simulink model "GFL_SMIB_Scan_LF_Investigation"  (R2024b)
settings: Solver=FixedStepAuto  StartTime=0  StopTime=200  FixedStep=Ts  RelTol=1e-3
PreLoadFcn:
  | FS_Frequency=csvread('Frequency_Sweep.csv',1,0); run lpf_param.m;
InitFcn:
  | FS_Frequency=csvread('Frequency_Sweep.csv',1,0); run lpf_param.m;
StartFcn:
  | FS_Frequency=csvread('Frequency_Sweep.csv',1,0); run lpf_param.m;
StopFcn:
  | run Bode_Draw.m
values from neighbouring files (symbols this model uses):
  D = zeros(6,4)    [TheoreticalImpedancePlot.m]    (also in TheoreticalImpedancePlotGFL.m = zeros(5,4))
  Fbase = 50    [lpf_param.m]
  fpll = 0.1    [lpf_param.m]
  k_lpf = 0.707    [lpf_param.m]
  wc_lpf = 2*pi*fc_lpf    (= 0.628318530718)    [lpf_param.m]
  x_e = [i_d; i_q; i_d_i; i_q_i; v_d_i; v_q_i; theta; v_dc; v_dc_i; i; i_i; v_lk; p_sum_i; p_lk_i]    [InterlinkAcDcB2B.m]
undefined symbols (not defined in the file or in its folder): ApparatusDiscreDamping, ApparatusPara, ApparatusPowerFlow, ApparatusType, DiscIntNeverNeededParam, OtherInputs, PowerFlow, Sbase, Ts, Vbase, Wbase, Ybase, Zbase
libraries: SimplusGT x10, discretizing x8, dspindex x4, spsGroundLib x3, simulink x3, spsControlledCurrentSourceLib x3, spsCurrentMeasurementLib x3, spsVoltageMeasurementLib x3, spsControlledVoltageSourceLib x3, spsThreePhaseSeriesRLCBranchLib x2, dspsnks4 x2, spsThreePhaseVIMeasurementLib x2
(part 2 of 2)

== matlab function GFL_SMIB_Scan_LF_Investigation/Frequency_Sweep/Frequency Sweep ==
  data: EN input; Perturb_DQ output; ResponseDQ input size=[1 6]; FreqSet input; FreqTest input; OutAmp input; Fs input; AmpGain input; xD input; FSResult output; FreqPoint output; RecordTrigger output; xD1 output; End output; CycleEnd output
function [Perturb_DQ, FSResult, FreqPoint, RecordTrigger, xD1, End, CycleEnd] = fcn(EN,ResponseDQ, FreqSet, FreqTest, OutAmp, Fs, AmpGain, xD)
% This function performs online frequency scanning using a state machine. 
%   - D and Q axis perturbations at specified frequencies
%   - The system response measured (Voltage and Currents)
%   - System admittance, Apparatus Admittance and Grid admittance are
%   calculated
% This current version uses a fixed window to detect whether steady state
% has been reached for each frequency point.
%
% Inputs:
%   EN          : Enable signal (1 to run, 0 to reset)
%   ResponseDQ  : 1x6 vector of system responses [ID, IQ, VAD, VAQ, VGD, VGQ]
%   FreqSet     : Vector of frequencies to apply perturbation (Hz)
%   FreqTest    : Vector of frequencies to analyze (DFT) (Hz)
%   OutAmp      : Vector of perturbation amplitudes for each frequency
%   Fs          : Sampling frequency (Hz)
%   AmpGain     : Global gain for perturbation amplitude
%   xD          : State vector (storage between calls)
%
% Outputs:
%   Perturb_DQ    : [OutVD, OutVQ] perturbation signal to inject
%   FSResult      : 2x6 complex vector of 2x2 admittances [Ysys, YA, YG]
%   FreqPoint     : The current frequency being tested
%   RecordTrigger : A one-sample pulse (==1) when a new result is calculated
%   xD1           : Updated state vector for the next time step
%   End           : Boolean Simulation End 
%
% ------------------- Tuning: Steady-state detector ---------------------- %
% These parameters control the sensitivity and speed of the steady-state detector.
MIN_CYCLES_WINDOWS = 1;    % always do at least one full test cycle before checking
MAX_CYCLES_WINDOWS = 20;   % safety cap to avoid hanging if state never stabilizes
TOL_MAG    = 1e-3;         % relative magnitude tolerance for steady-state (0.1%)
TOL_PHASE  = 1*pi/180;     % phase tolerance (radians) (~1 deg)
STABLE_K   = 1;            % consecutive stable cycles required to confirm steady state
EPS        = 1e-12;        % small number to prevent division by zero
CYCLES = 5;                % number of cycles to use for each fixed DFT window
% -------------------Initialise Outputs-----------------------------------%
% Pre-allocate output matrices for admittances
YA        = complex(zeros(2,2)); % Admittance YA = -I / VA
YG        = complex(zeros(2,2)); % Admittance YG = I / VG
Ysys      = complex(zeros(2,2)); % System Admittance Ysys = I / V_perturb
FSResult  = complex(zeros(2,6)); % Final result matrix [Ysys, YA, YG]
RecordTrigger = 0;               % Output trigger pulse
End = 0;                         % Simulation End Boolean
CycleEnd = 0;
% ------------------- Read States ----------------------------------------%
% 'xD' stores the function's internal state between simulation steps.
CaseK = xD(1);    % Current state in the state machine (0, 1, 2, 3, 9)
Ns    = xD(2);    % Number of samples for perturbation signal generation
Nt    = xD(3);    % Number of samples for DFT analysis window
n     = xD(4);    % Current sample counter within a window (1 to Nt)
kc    = xD(5);    % Current frequency index (points to FreqSet(kc))
OutVD = xD(6);    % Current D-axis perturbation output
OutVQ = xD(7);    % Current Q-axis perturbation output
% Sums for DFT accumulation [ID, IQ, VAD, VAQ, VGD, VGQ]
% These are complex accumulators for the 6 response signals.
Sum = complex([xD(8)+1i*xD(9),  xD(10)+1i*xD(11), ...
               xD(20)+1i*xD(21), xD(22)+1i*xD(23), ...
               xD(32)+1i*xD(33), xD(34)+1i*xD(35)]);
% Final DFT results after D-axis sweep [ID, IQ, VAD, VAQ, VGD, VGQ]
FinalD = complex([xD(12)+1i*xD(13),  xD(14)+1i*xD(15), ...
                  xD(24)+1i*xD(25),  xD(26)+1i*xD(27), ...
                  xD(36)+1i*xD(37),  xD(38)+1i*xD(39)]).'; % Transpose to 6x1
% Final DFT results after Q-axis sweep [ID, IQ, VAD, VAQ, VGD, VGQ]
FinalQ = complex([xD(16)+1i*xD(17),  xD(18)+1i*xD(19), ...
                  xD(28)+1i*xD(29),  xD(30)+1i*xD(31), ...
                  xD(40)+1i*xD(41),  xD(42)+1i*xD(43)]).'; % Transpose to 6x1
% --- Legacy TWait(44) removed ---
% Steady-state detector states (shifted down by 1)
cycCount     = xD(44);     % Number of test cycles completed at this frequency
stableCount  = xD(45);     % Number of consecutive stable cycles
PrevRe       = [xD(46) xD(47) xD(48) xD(49) xD(50) xD(51)]; % Real part of previous DFT
PrevIm       = [xD(52) xD(53) xD(54) xD(55) xD(56) xD(57)]; % Imag part of previous DFT
Prev         = complex(PrevRe(:), PrevIm(:));   % 6x1 complex vector of previous DFT results
% Get total number of frequencies to test
FrequencyNum = numel(FreqSet);
% --- Safety Check ---
% Ensure gain is not zero, which would cause division by zero later
if AmpGain==0 || (kc>=1 && kc<=FrequencyNum && OutAmp(kc)==0)
    error('AmpGain and OutAmp(kc) must be non-zero');
end
% Reshape response input to a 1x6 row vector for easier matrix math
Resp = reshape(ResponseDQ,1,6);

%% Main Loop
if EN==0
    % If Enable is low, reset the perturbation outputs
    OutVD=0;
    OutVQ=0;
    % Note: State variables are NOT reset here, they are reset in Case 0
    % when EN goes high.
else
    % --- State Machine ---
    switch CaseK
        case 0  % State 0: Initialization
            RecordTrigger = 0; % Ensure trigger is low
            kc = 1;            % Start with the first frequency
            CaseK = 1;         % Move to setup state
            CycleEnd = 0;
        case 1  % State 1: Setup for new frequency
            if kc > FrequencyNum
                % If frequency index is past the end of the list, sweep is done
                OutVD=0; OutVQ=0; % Turn off perturbation
                CaseK = 9;       % Move to 'finished' state
            else
                % --- Prepare for a new frequency sweep ---
                Sum(:)=0;  % Reset DFT accumulators
                % Calculate number of samples for perturbation generation (Ns)
                % and DFT analysis (Nt) based on Fs, Freq, and CYCLES
                Ns = max(1, round(Fs/FreqSet(kc)*CYCLES));
                Nt = max(1, round(Fs/FreqTest(kc)*CYCLES));
                OutVD=0; OutVQ=0; % Ensure perturbation is off during setup
                n = 1;            % Reset sample counter
                % Reset steady-state detector variables
                cycCount = 0;
                stableCount = 0;
                Prev(:) = 0;
                CaseK = 2;         % Move to D-axis perturbation state
            end
        case 2   % State 2: D-axis perturbation and analysis
            % Generate D-axis sinusoidal perturbation
            OutVD = OutAmp(kc)*sin(2*pi*CYCLES*n/Ns)*AmpGain;
            OutVQ = 0;
            % Calculate DFT complex phasor for this sample
            ang = 2*pi*CYCLES*(n-1)/Nt;
            ph  = sin(ang) + 1i*cos(ang);
            % Accumulate the DFT sum (dot product of response and phasor)
            % % --------- Hanning window weight for this sample ---------
            % if Nt > 1
            %     w_n = 0.5 - 0.5*cos(2*pi*(n-1)/(Nt-1));
            % else
            %     w_n = 1;
            % end
            % Resp_w = Resp * w_n;
            % 
            % % Accumulate the DFT sum (windowed)
            % Sum = Sum + Resp_w * ph;
            Sum = Sum + Resp * ph;
            if n < Nt
                % If window is not full, increment sample counter
                n = n + 1;
            else
                % --- One test cycle completed on D-axis ---
                % Scale the accumulated sum to get the DFT phasor
                scale  = 2*FreqSet(kc)/CYCLES/Fs; % DFT scaling factor
                Curr   = scale*Sum.';     % 6x1 complex phasor result
                if cycCount >= 1
                    % --- Steady-State Check (if not the first cycle) ---
                    % Compare current result (Curr) vs. previous (Prev)
                    % Calculate relative magnitude difference
                    dmag   = abs(abs(Curr) - abs(Prev)) ./ max(abs(Curr), EPS);
                    % Calculate phase difference
                    dphase = angle(Curr) - angle(Prev);
                    % Wrap phase difference to [-pi, pi]
                    dphase = atan2(sin(dphase), cos(dphase));
                    % Check if all 6 signals are stable within tolerance
                    isStable = all(dmag <= TOL_MAG) && all(abs(dphase) <= TOL_PHASE);
                    if isStable
                        stableCount = stableCount + 1; % Increment stable counter
                    else
                        stableCount = 0; % Reset if any signal is unstable
                    end
                end
                Prev      = Curr;         % Store current result for next comparison
                cycCount  = cycCount + 1; % Increment total cycle counter
                % --- Decision: Move on or repeat? ---
                if (cycCount >= MIN_CYCLES_WINDOWS && stableCount >= STABLE_K) || (cycCount >= MAX_CYCLES_WINDOWS)
                    % Condition 1: Min cycles done AND stable count reached
                    % Condition 2: Max cycles limit reached

                    % Accept this result as steady-state for D-axis
                    FinalD = Prev;
                    % Prepare for Q-axis sweep
                    Sum(:) = 0; n = 1; % Reset accumulators and counter
                    cycCount = 0; stableCount = 0; % Reset detector
                    Prev(:)  = 0;
                    CaseK = 3;         % Move to Q-axis state
                    CycleEnd = 1;
                else
                    % Not stable yet, run another test cycle
                    Sum(:) = 0; n = 1;   % Reset for another D-axis cycle
                    % Stay in CaseK = 2
                end
            end
        case 3   % State 3: Q-axis perturbation and analysis
            % This state is analogous to Case 2, but for the Q-axis.
            CycleEnd = 0;
            OutVD = 0;
            OutVQ = OutAmp(kc)*sin(2*pi*CYCLES*n/Ns)*AmpGain;
            % Calculate DFT complex phasor
            ang = 2*pi*CYCLES*(n-1)/Nt;
            ph  = sin(ang) + 1i*cos(ang);
            % Accumulate the DFT sum (dot product of response and phasor)
            % % --------- Hanning window weight for this sample ---------
            % if Nt > 1
            %     w_n = 0.5 - 0.5*cos(2*pi*(n-1)/(Nt-1));
            % else
            %     w_n = 1;
            % end
            % Resp_w = Resp * w_n;

            % Accumulate the DFT sum (windowed)
            % Sum = Sum + Resp_w * ph;
            Sum = Sum + Resp * ph;
            if n < Nt
                % If window is not full, increment sample counter
                n = n + 1;
            else
                % --- One test cycle completed on Q-axis ---
                scale  = 2*FreqSet(kc)/CYCLES/Fs; % DFT scaling
                Curr   = scale*Sum.';     % 6x1 complex phasor
                % --- Steady-State Check ---
                if cycCount >= 1
                    dmag   = abs(abs(Curr) - abs(Prev)) ./ max(abs(Curr), EPS);
                    dphase = angle(Curr) - angle(Prev);
                    dphase = atan2(sin(dphase), cos(dphase));
                    isStable = all(dmag <= TOL_MAG) && all(abs(dphase) <= TOL_PHASE);
                    if isStable
                        stableCount = stableCount + 1;
                    else
                        stableCount = 0;
                    end
                end
                Prev      = Curr;
                cycCount  = cycCount + 1;
                % --- Decision: Finalize or repeat? ---
                if (cycCount >= MIN_CYCLES_WINDOWS && stableCount >= STABLE_K) || (cycCount >= MAX_CYCLES_WINDOWS)
                    % Steady state reached for Q-axis
                    FinalQ = Prev;
                    % --- Calculate Admittances ---
                    % Build 2x2 matrices from the 6x1 D and Q result vectors
                    % I = [I_d_from_Vd, I_d_from_Vq; I_q_from_Vd, I_q_from_Vq]
                    I  = [FinalD(1), FinalQ(1);  FinalD(2), FinalQ(2)];
                    VA = [FinalD(3), FinalQ(3);  FinalD(4), FinalQ(4)];
                    VG = [FinalD(5), FinalQ(5);  FinalD(6), FinalQ(6)];
                    % Calculate admittance matrices using pseudo-inverse (pinv)
                    % for numerical stability.
                    % Y = I * V^-1
                    YA  = -I * pinv(VA);  % Note the negative sign
                    YG  = I * pinv(VG);

                    % Ysys is calculated relative to the known perturbation amplitude
                    % V_perturb = [Amp, 0; 0, Amp] (assuming same D/Q amp)
                    % Ysys = I * V_perturb^-1
                    Ysys = -I/(OutAmp(kc)*AmpGain);
                    % Set trigger pulse high for one sample
                    RecordTrigger = 1;
                    CycleEnd = 1;

                    % --- Advance to next frequency ---
                    kc = kc + 1;
                    if kc > FrequencyNum
                        % Finished all frequencies
                        CaseK = 9;
                    else
                        % Prepare for next frequency
                        Sum(:)=0; n=1; cycCount=0; stableCount=0; Prev(:)=0;
                        CaseK = 1; % Go back to setup state
                    end
                else
                    % Not stable, run another Q-axis test cycle
                    Sum(:) = 0; n = 1;
                    % Stay in CaseK = 3
                end
            end
        case 9  % State 9: Finished
            % Sweep is complete. Hold outputs at 0.
            OutVD=0;
            OutVQ=0;
            % The state machine will stay here until EN=0.
    end
end
%% Set Outputs
% Pack all internal states back into the 'xD1' state vector
% This ensures they are saved for the next function call.

xD1 = zeros(1,57);   % Initialize output state vector (new length 57)
xD1(1:7)   = [CaseK, Ns, Nt, n, kc, OutVD, OutVQ]; % Main states

% Pack DFT sums (complex -> 2 reals)
xD1(8:11)  = [real(Sum(1)), imag(Sum(1)), real(Sum(2)), imag(Sum(2))]; % ID, IQ
xD1(20:23) = [real(Sum(3)), imag(Sum(3)), real(Sum(4)), imag(Sum(4))]; % VAD, VAQ
xD1(32:35) = [real(Sum(5)), imag(Sum(5)), real(Sum(6)), imag(Sum(6))]; % VGD, VGQ

% Pack Final D-axis results
xD1(12:15) = [real(FinalD(1)), imag(FinalD(1)), real(FinalD(2)), imag(FinalD(2))];
xD1(24:27) = [real(FinalD(3)), imag(FinalD(3)), real(FinalD(4)), imag(FinalD(4))];
xD1(36:39) = [real(FinalD(5)), imag(FinalD(5)), real(FinalD(6)), imag(FinalD(6))];

% Pack Final Q-axis results
xD1(16:19) = [real(FinalQ(1)), imag(FinalQ(1)), real(FinalQ(2)), imag(FinalQ(2))];
xD1(28:31) = [real(FinalQ(3)), imag(FinalQ(3)), real(FinalQ(4)), imag(FinalQ(4))];
xD1(40:43) = [real(FinalQ(5)), imag(FinalQ(5)), real(FinalQ(6)), imag(FinalQ(6))];

% --- TWait(44) removed, states shifted ---
% Pack steady-state detector states
xD1(44) = cycCount;
xD1(45) = stableCount;
xD1(46:51) = real(Prev).';   % 6 real parts
xD1(52:57) = imag(Prev).';   % 6 imaginary parts

% --- Assign final function outputs ---
Perturb_DQ = [OutVD, OutVQ]; % Perturbation signal
if kc>0 && EN==1
    % Reshape 2x2 matrices into a 2x6 complex row vector for output
    FSResult = [Ysys, YA, YG];

    % Decide which frequency index to report:
    % - When RecordTrigger==1, a result for the *previous* kc was just finalized,
    %   but kc has already been incremented. Report kc-1 in that case.
    % - Otherwise, report the current kc being processed.
    if RecordTrigger==1
        idx = kc - 1;
    else
        idx = kc;
    end

    % Clamp idx to valid range [1, FrequencyNum]
    if FrequencyNum >= 1
        idx = max(1, min(idx, FrequencyNum));
        FreqPoint = FreqSet(idx);
    else
        FreqPoint = 0;
    end
    End = double(CaseK==9);
else
    % If disabled or not started, output zeros
    FSResult(:) = 0;
    FreqPoint   = 0;
    End         = 0;             
end
end
